simulink model "TRIAD"  (R2019a)
settings: Solver=VariableStepAuto  StartTime=0.0  StopTime=10.0  RelTol=1e-3
libraries: vrlib x8, sharedtransform x1
settings Model: Creator=Owner  LastModifiedBy=Owner

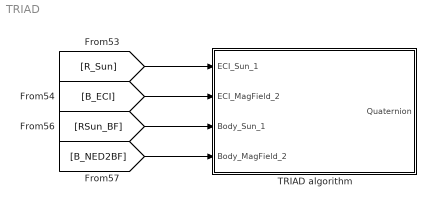
== system TRIAD ==
  TRIAD algorithm : Subsystem
  wires:
  [B_ECI] -> TRIAD algorithm/2(ECI_MagField_2)
  [R_Sun] -> TRIAD algorithm/1(ECI_Sun_1)
  [B_NED2BF] -> TRIAD algorithm/4(Body_MagField_2)
  [RSun_BF] -> TRIAD algorithm/3(Body_Sun_1)

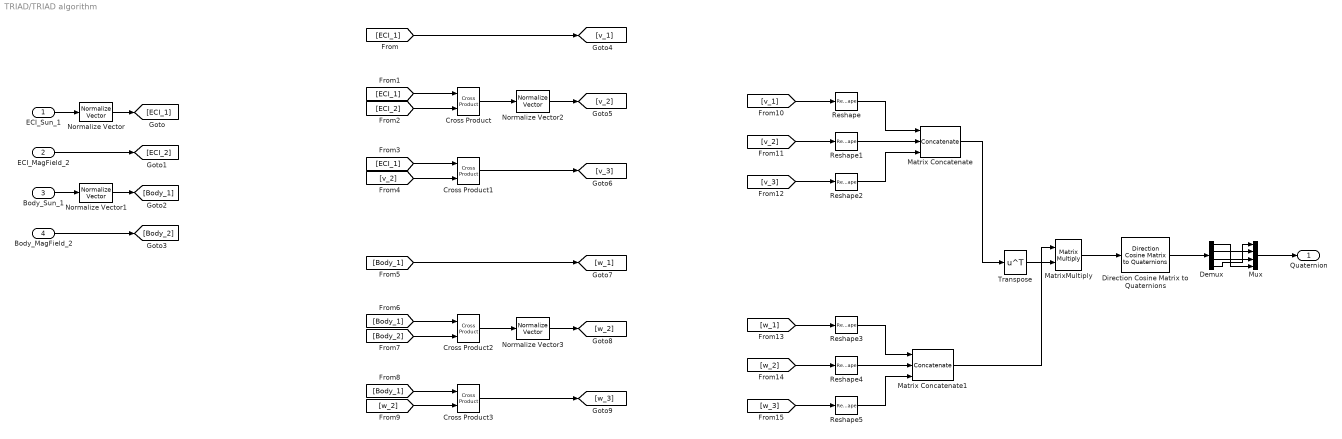
== system TRIAD/TRIAD algorithm ==
  ECI_Sun_1 : Inport
  ECI_MagField_2 : Inport  Port=2
  Body_Sun_1 : Inport  Port=3
  Body_MagField_2 : Inport  Port=4
  Cross Product{,1..3} (4 alike) : vrlib/Utilities/Cross Product
  Demux : Demux
  Direction Cosine Matrix to Quaternions : sharedtransform/Direction Cosine Matrix  to Quaternions  aMode=0  action=None  tolerance=eps(2)
      settings: SourceProductBaseCode=AE,PW,MT,UV,VE,VP
  Matrix Concatenate : Concatenate  NumInputs=3  Mode=Multidimensional array  ConcatenateDimension=2
  Matrix Concatenate1 : Concatenate  NumInputs=3  Mode=Multidimensional array  ConcatenateDimension=2
  MatrixMultiply : Product  Multiplication=Matrix(*)
  Mux : Mux
  Normalize Vector{,1..3} (4 alike) : vrlib/Utilities/Normalize Vector  maxzero=0
  Reshape{,1..5} (6 alike) : Reshape  OutputDimensionality=Column vector (2-D)
  Transpose : Math  Operator=transpose  SaturateOnIntegerOverflow=on
  Quaternion : Outport  VectorParamsAs1DForOutWhenUnconnected=on
  wires:
  Cross Product/1 -> Normalize Vector2/1
  Reshape1/1 -> Matrix Concatenate/2
  [ECI_1] -> Cross Product1/1
  Body_MagField_2/1 -> [Body_2]
  ECI_MagField_2/1 -> [ECI_2]
  Reshape2/1 -> Matrix Concatenate/3
  Cross Product3/1 -> [w_3]
  [ECI_1] -> [v_1]
  Normalize Vector1/1 -> [Body_1]
  [w_1] -> Reshape3/1
  Body_Sun_1/1 -> Normalize Vector1/1
  [v_2] -> Reshape1/1
  ECI_Sun_1/1 -> Normalize Vector/1
  [Body_1] -> Cross Product2/1
  [ECI_1] -> Cross Product/1
  Normalize Vector3/1 -> [w_2]
  Cross Product2/1 -> Normalize Vector3/1
  [Body_1] -> Cross Product3/1
  Cross Product1/1 -> [v_3]
  Normalize Vector/1 -> [ECI_1]
  MatrixMultiply/1 -> Direction Cosine Matrix to Quaternions/1
  Normalize Vector2/1 -> [v_2]
  [ECI_2] -> Cross Product/2
  Reshape3/1 -> Matrix Concatenate1/1
  [v_2] -> Cross Product1/2
  [Body_1] -> [w_1]
  [w_3] -> Reshape5/1
  [v_3] -> Reshape2/1
  [v_1] -> Reshape/1
  [w_2] -> Cross Product3/2
  [Body_2] -> Cross Product2/2
  [w_2] -> Reshape4/1
  Reshape5/1 -> Matrix Concatenate1/3
  Reshape/1 -> Matrix Concatenate/1
  Reshape4/1 -> Matrix Concatenate1/2
  Matrix Concatenate1/1 -> MatrixMultiply/1
  Matrix Concatenate/1 -> Transpose/1
  Transpose/1 -> MatrixMultiply/2
  Direction Cosine Matrix to Quaternions/1 -> Demux/1
  Demux/1 -> Mux/4
  Demux/2 -> Mux/1
  Demux/3 -> Mux/2
  Demux/4 -> Mux/3
  Mux/1 -> Quaternion/1
